simulink model "PandID"  (R2019b)
settings: Solver=VariableStepAuto  StartTime=0.0  StopTime=50  RelTol=1e-3
values from neighbouring files (symbols this model uses):
  L_area = 1    [AFCP_sim.m]
  P_area = 1    [AFCP_sim.m]
  PressureUnit = 1/6894.76    (= 0.000145037680789)    [AFCP_sim.m]
  R_area = 1    [AFCP_sim.m]
  Valve_signal_Unit = 0.00064516    [AFCP_sim.m]
libraries: fl_lib x96, nesl_utility x62, SimscapeFluids_lib x15, simulink x4
(part 1 of 2)
settings Model: OrderedModelArguments=off  Creator=abhig  LastModifiedBy=abhig
settings SFSimCC: SimUserSources=init.c main.c seq.c  SimParseCustomCode=off
settings SFSimCC: SimCustomHeaderCode=|
  | #include "headers.h"
  | #include "init.h"
  | #include "macros.h"
  | #include "seq.h"
settings SFSimCC: SimUserIncludeDirs=|
  | C:\Users\abhig\OneDrive\Desktop\simulation\AFCP_SIMULINK\simulink_test\flightCode\src
  | 
  | C:\Users\abhig\OneDrive\Desktop\simulation\AFCP_SIMULINK\simulink_test\flightCode\include

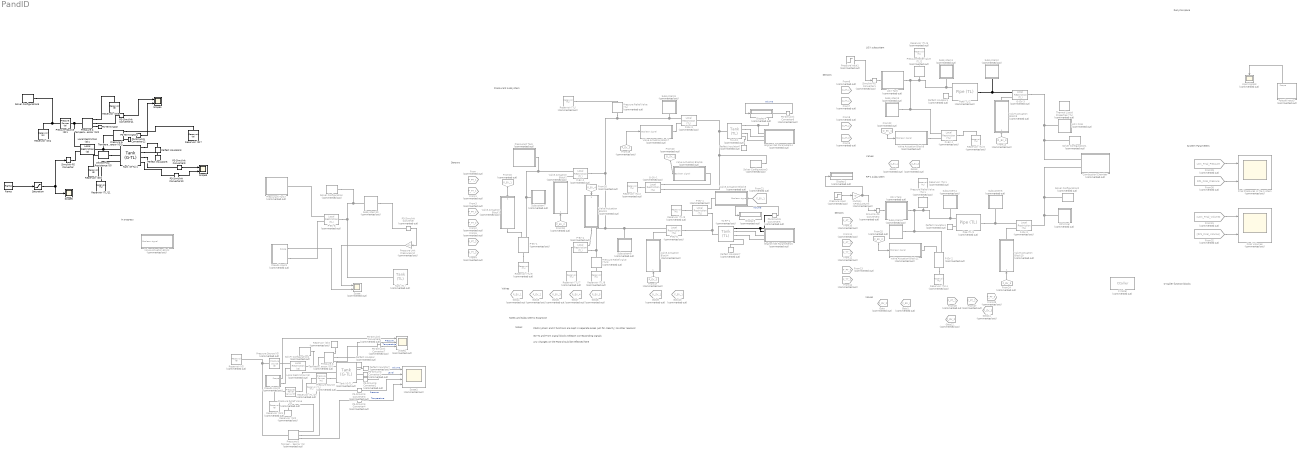
== system PandID ==
  note: System Parameters
  note: In progress
  note: Sensors
  note: Valves
  note: Valves
  note: Sensors
  note: Valves
  note: Sensors
  note: P&ID system and C functions are kept in seperate areas just for clearity; No other reasons!
  note: Notes:
  note: Recycle space
  note: Notes and Subsystems expansion
  note: RP-1 subsystem
  note: Pressurant subsystem
  note: LOX subsystem
  note: C-Caller function blocks
  note: Go-To and From signal blocks teleport corresponding signals
  note: Any changes on the P&ID should be reflected here
  C Caller : CCaller  Commented=on  FunctionName=init  PortSpecificationStruct="%)30     .    , (   8    (     @         %    \"     $    !     0         %  0 \"0    $    _    07)G3F%M90  4&]R=$YA;64 4V-O<&4     26YD97@     5'EP90      4VEZ90      27-';&]B86P   X   !     !@    @    $          4    (     0    D    !         !     )    9FEL95]N86UE          X   !     !@    @    $          4    (     0    D    !         !     )    9FEL95]N86UE          X    X    !@    @    $          4    (     0    8    !         !     &    3W5T<'5T   .    .     8    (    !@         %    \"     $    !     0         )    \"               #@   #     &    \"     0         !0    @    !    !     $         $  $ &EN=#@.    ,     8    (    !          %    \"     $    \"     0         0  ( +3$   X    P    !@    @    ) @        4    (     0    $    !          (  0"
  Combustion Chamber : Subsystem  Commented=on
      mask Display: image('$imagefile'); % Use "Edit Image" on toolstrip to change.
  Display1 : Display  Commented=on
  Display4 : Display  Commented=on
  Display5 : Display  Commented=on
  Engine Inlet Parameters4 : Subsystem  Commented=on
  Engine Inlet Parameters5 : Subsystem  Commented=on
  F-EV-1 : fl_lib/Thermal Liquid/Elements/Local Restriction (TL)  Commented=on  restriction_type=foundation.enum.restriction_type.variable  restriction_area=0.001 m^2  min_area=1e-5 m^2  max_area=0.005 m^2  area=0.01 m^2  Cd=0.64  pressure_recovery=simscape.enum.onoff.on  Re_c=12
      settings: SourceProductName=Simscape  SourceProductBaseCode=SS  InternalSimscapePortConfiguration="{\"Bottom\":[],\"Left\":[{\"id\":\"A\",\"label\":\"A\",\"type\":\"foundation.thermal_liquid.thermal_liquid\"},{\"id\":\"area_in\",\"label\":\"AR\",\"type\":\"input\"}],\"Right\":[{\"id\":\"B\",\"label\":\"B\",\"type\":\"foundation.thermal_liquid.thermal_liquid\"}],\"Top\":[]}"
  F-EV-2 : fl_lib/Thermal Liquid/Elements/Local Restriction (TL)  Commented=on  restriction_type=foundation.enum.restriction_type.variable  restriction_area=0.001 m^2  min_area=R_area*0.01 in^2  max_area=R_area*0.99 in^2  area=R_area in^2  Cd=0.64  pressure_recovery=simscape.enum.onoff.on  Re_c=12
      settings: SourceProductName=Simscape  SourceProductBaseCode=SS  InternalSimscapePortConfiguration="{\"Bottom\":[],\"Left\":[{\"id\":\"A\",\"label\":\"A\",\"type\":\"foundation.thermal_liquid.thermal_liquid\"},{\"id\":\"area_in\",\"label\":\"AR\",\"type\":\"input\"}],\"Right\":[{\"id\":\"B\",\"label\":\"B\",\"type\":\"foundation.thermal_liquid.thermal_liquid\"}],\"Top\":[]}"
  F-EV-3 : fl_lib/Thermal Liquid/Elements/Local Restriction (TL)  Commented=on  restriction_type=foundation.enum.restriction_type.variable  restriction_area=0.001 m^2  min_area=1e-5 in^2  max_area=R_area/2 in^2  area=R_area in^2  Cd=0.64  pressure_recovery=simscape.enum.onoff.on  Re_c=12
      settings: SourceProductName=Simscape  SourceProductBaseCode=SS  InternalSimscapePortConfiguration="{\"Bottom\":[],\"Left\":[{\"id\":\"A\",\"label\":\"A\",\"type\":\"foundation.thermal_liquid.thermal_liquid\"},{\"id\":\"area_in\",\"label\":\"AR\",\"type\":\"input\"}],\"Right\":[{\"id\":\"B\",\"label\":\"B\",\"type\":\"foundation.thermal_liquid.thermal_liquid\"}],\"Top\":[]}"
  Final Pressures in the system : Scope  Commented=on  NumInputPorts=2
  Final Volumes : Scope  Commented=on  NumInputPorts=2
  From : From  Commented=on  GotoTag=P_PT_1  TagVisibility=global
  From1 : From  Commented=on  GotoTag=P_TT_1  TagVisibility=global
  From10 : From  Commented=on  GotoTag=F_PT_1  TagVisibility=global
  From11 : From  Commented=on  GotoTag=F_PT_2  TagVisibility=global
  From12 : From  Commented=on  GotoTag=F_TT_2  TagVisibility=global
  From13 : From  Commented=on  GotoTag=F_PT_3  TagVisibility=global
  From14 : From  Commented=on  GotoTag=F_TT_3  TagVisibility=global
  From15 : From  Commented=on  GotoTag=P_EV_1  TagVisibility=global
  From16 : From  Commented=on  GotoTag=P_EV_4  TagVisibility=global
  From17 : From  Commented=on  GotoTag=P_EV_5  TagVisibility=global
  From18 : From  Commented=on  GotoTag=P_EV_2  TagVisibility=global
  From19 : From  Commented=on  GotoTag=P_EV_3  TagVisibility=global
  From2 : From  Commented=on  GotoTag=P_TT_2  TagVisibility=global
  From20 : From  Commented=on  GotoTag=O_SV_1  TagVisibility=global
  From21 : From  Commented=on  GotoTag=F_EV_1  TagVisibility=global
  From22 : From  Commented=on  GotoTag=O_EV_1  TagVisibility=global
  From23 : From  Commented=on  GotoTag=O_EV_3  TagVisibility=global
  From24 : From  Commented=on  GotoTag=F_EV_3  TagVisibility=global
  From25 : From  Commented=on  GotoTag=F_EV_2  TagVisibility=global
  From26 : From  Commented=on  GotoTag=F_PT_1  TagVisibility=global
  From27 : From  Commented=on  GotoTag=F_PT_2  TagVisibility=global
  From28 : From  Commented=on  GotoTag=F_PT_3  TagVisibility=global
  From29 : From  Commented=on  GotoTag=LOX_Final_Pressure
  From3 : From  Commented=on  GotoTag=P_PT_2  TagVisibility=global
  From30 : From  Commented=on  GotoTag=RP1_Final_Pressure
  From31 : From  Commented=on  GotoTag=LOX_Final_Volume
  From32 : From  Commented=on  GotoTag=RP1_Final_Volume
  From4 : From  Commented=on  GotoTag=P_TT_3  TagVisibility=global
  From5 : From  Commented=on  GotoTag=P_PT_3  TagVisibility=global
  From6 : From  Commented=on  GotoTag=O_PT_1  TagVisibility=global
  From7 : From  Commented=on  GotoTag=O_TT_1  TagVisibility=global
  From8 : From  Commented=on  GotoTag=O_PT_2  TagVisibility=global
  From9 : From  Commented=on  GotoTag=O_PT_3  TagVisibility=global
  Goto : Goto  Commented=on  GotoTag=F_EV_2  TagVisibility=global
  Goto1 : Goto  Commented=on  GotoTag=F_EV_3  TagVisibility=global
  Goto10 : Goto  Commented=on  GotoTag=F_EV_1  TagVisibility=global
  Goto11 : Goto  Commented=on  GotoTag=F_EV_3  TagVisibility=global
  Goto12 : Goto  Commented=on  GotoTag=F_EV_2  TagVisibility=global
  Goto2 : Goto  Commented=on  GotoTag=O_EV_1  TagVisibility=global
  Goto3 : Goto  Commented=on  GotoTag=O_EV_3  TagVisibility=global
  Goto4 : Goto  Commented=on  GotoTag=P_EV_1  TagVisibility=global
  Goto5 : Goto  Commented=on  GotoTag=P_EV_2  TagVisibility=global
  Goto6 : Goto  Commented=on  GotoTag=P_EV_3  TagVisibility=global
  Goto7 : Goto  Commented=on  GotoTag=P_EV_4  TagVisibility=global
  Goto8 : Goto  Commented=on  GotoTag=P_EV_5  TagVisibility=global
  Goto9 : Goto  Commented=on  GotoTag=O_SV_1  TagVisibility=global
  Infinite Flow Resistance (G) : fl_lib/Gas/Elements/Infinite Flow Resistance (G)  p_specify=off  p_priority=None  p=0 MPa  p_nominal_specify=off  p_nominal_unit=MPa  p_nominal_value=1  T_specify=off  T_priority=None  T=0 K  T_nominal_specify=off  T_nominal_unit=K  T_nominal_value=1
      settings: SourceProductName=Simscape  SourceProductBaseCode=SS  InternalSimscapePortConfiguration="{\"Bottom\":[],\"Left\":[{\"id\":\"A\",\"label\":\"A\",\"type\":\"foundation.gas.gas\"}],\"Right\":[{\"id\":\"B\",\"label\":\"B\",\"type\":\"foundation.gas.gas\"}],\"Top\":[]}"
  Input signal3 : Scope  Commented=on
  LOX Final : Subsystem  Commented=on
      mask Display: image('$imagefile'); % Use "Edit Image" on toolstrip to change.
  LOX Tank : Subsystem  Commented=on
      mask Display: image('$imagefile'); % Use "Edit Image" on toolstrip to change.
  Local Restriction (G) : fl_lib/Gas/Elements/Local Restriction (G)  Commented=on  restriction_type=foundation.enum.restriction_type.variable  restriction_area=1e-3 m^2  min_area=1e-10 m^2  max_area=0.005 m^2  area=0.01 m^2  Cd=0.64  B_lam=0.999
      settings: SourceProductName=Simscape  SourceProductBaseCode=SS  InternalSimscapePortConfiguration="{\"Bottom\":[],\"Left\":[{\"id\":\"A\",\"label\":\"A\",\"type\":\"foundation.gas.gas\"},{\"id\":\"area_in\",\"label\":\"AR\",\"type\":\"input\"}],\"Right\":[{\"id\":\"B\",\"label\":\"B\",\"type\":\"foundation.gas.gas\"}],\"Top\":[]}"
  Local Restriction (G)1 : fl_lib/Gas/Elements/Local Restriction (G)  restriction_type=foundation.enum.restriction_type.variable  restriction_area=1e-3 m^2  min_area=1e-10 m^2  max_area=0.005 m^2  area=0.01 m^2  Cd=0.64  B_lam=0.999
      settings: SourceProductName=Simscape  SourceProductBaseCode=SS  InternalSimscapePortConfiguration="{\"Bottom\":[],\"Left\":[{\"id\":\"A\",\"label\":\"A\",\"type\":\"foundation.gas.gas\"},{\"id\":\"area_in\",\"label\":\"AR\",\"type\":\"input\"}],\"Right\":[{\"id\":\"B\",\"label\":\"B\",\"type\":\"foundation.gas.gas\"}],\"Top\":[]}"
  Multiply : Gain  Commented=on  Gain=1/PressureUnit
  O-EV-1 : fl_lib/Thermal Liquid/Elements/Local Restriction (TL)  Commented=on  restriction_type=foundation.enum.restriction_type.variable  restriction_area=0.001 m^2  min_area=1e-5 m^2  max_area=0.005 m^2  area=L_area in^2  Cd=0.64  pressure_recovery=simscape.enum.onoff.on  Re_c=12
      settings: SourceProductName=Simscape  SourceProductBaseCode=SS  InternalSimscapePortConfiguration="{\"Bottom\":[],\"Left\":[{\"id\":\"A\",\"label\":\"A\",\"type\":\"foundation.thermal_liquid.thermal_liquid\"},{\"id\":\"area_in\",\"label\":\"AR\",\"type\":\"input\"}],\"Right\":[{\"id\":\"B\",\"label\":\"B\",\"type\":\"foundation.thermal_liquid.thermal_liquid\"}],\"Top\":[]}"
  O-EV-3 : fl_lib/Thermal Liquid/Elements/Local Restriction (TL)  Commented=on  restriction_type=foundation.enum.restriction_type.variable  restriction_area=0.001 m^2  min_area=1e-5 m^2  max_area=0.005 m^2  area=L_area in^2  Cd=0.64  pressure_recovery=simscape.enum.onoff.on  Re_c=12
      settings: SourceProductName=Simscape  SourceProductBaseCode=SS  InternalSimscapePortConfiguration="{\"Bottom\":[],\"Left\":[{\"id\":\"A\",\"label\":\"A\",\"type\":\"foundation.thermal_liquid.thermal_liquid\"},{\"id\":\"area_in\",\"label\":\"AR\",\"type\":\"input\"}],\"Right\":[{\"id\":\"B\",\"label\":\"B\",\"type\":\"foundation.thermal_liquid.thermal_liquid\"}],\"Top\":[]}"
  O-SV-1 : fl_lib/Thermal Liquid/Elements/Local Restriction (TL)  Commented=on  restriction_type=foundation.enum.restriction_type.variable  restriction_area=0.001 m^2  min_area=1e-5 m^2  max_area=0.005 m^2  area=P_area in^2  Cd=0.64  pressure_recovery=simscape.enum.onoff.on  Re_c=12
      settings: SourceProductName=Simscape  SourceProductBaseCode=SS  InternalSimscapePortConfiguration="{\"Bottom\":[],\"Left\":[{\"id\":\"A\",\"label\":\"A\",\"type\":\"foundation.thermal_liquid.thermal_liquid\"},{\"id\":\"area_in\",\"label\":\"AR\",\"type\":\"input\"}],\"Right\":[{\"id\":\"B\",\"label\":\"B\",\"type\":\"foundation.thermal_liquid.thermal_liquid\"}],\"Top\":[]}"
  P-EV-{1..5} (5 alike) : fl_lib/Thermal Liquid/Elements/Local Restriction (TL)  Commented=on  restriction_type=foundation.enum.restriction_type.variable  restriction_area=0.001 m^2  min_area=1e-5 m^2  max_area=0.005 m^2  area=P_area in^2  Cd=0.64  pressure_recovery=simscape.enum.onoff.on  Re_c=12
      settings: SourceProductName=Simscape  SourceProductBaseCode=SS  InternalSimscapePortConfiguration="{\"Bottom\":[],\"Left\":[{\"id\":\"A\",\"label\":\"A\",\"type\":\"foundation.thermal_liquid.thermal_liquid\"},{\"id\":\"area_in\",\"label\":\"AR\",\"type\":\"input\"}],\"Right\":[{\"id\":\"B\",\"label\":\"B\",\"type\":\"foundation.thermal_liquid.thermal_liquid\"}],\"Top\":[]}"
  P-EV-6 : fl_lib/Thermal Liquid/Elements/Local Restriction (TL)  Commented=on  restriction_type=foundation.enum.restriction_type.variable  restriction_area=0.001 m^2  min_area=P_area*0.01 in^2  max_area=P_area*0.99 in^2  area=P_area in^2  Cd=0.64  pressure_recovery=simscape.enum.onoff.on  Re_c=12
      settings: SourceProductName=Simscape  SourceProductBaseCode=SS  InternalSimscapePortConfiguration="{\"Bottom\":[],\"Left\":[{\"id\":\"A\",\"label\":\"A\",\"type\":\"foundation.thermal_liquid.thermal_liquid\"},{\"id\":\"area_in\",\"label\":\"AR\",\"type\":\"input\"}],\"Right\":[{\"id\":\"B\",\"label\":\"B\",\"type\":\"foundation.thermal_liquid.thermal_liquid\"}],\"Top\":[]}"
  PS Terminator : fl_lib/Physical Signals/Sinks/PS Terminator
      settings: SourceProductName=Simscape
  PS Terminator1 : fl_lib/Physical Signals/Sinks/PS Terminator
      settings: SourceProductName=Simscape
  PS-Simulink Converter{,1..8} (9 alike) : nesl_utility/PS-Simulink Converter  Commented=on  PhysicalDomain=network_engine_domain  SubClassName=ps_output  LeftPortType=input  RightPortType=output  PseudoPeriodic=off  Frequencies=[]  Unit=inherit  AffineConversion=off
  PS-Simulink Converter{9..12} (4 alike) : nesl_utility/PS-Simulink Converter  PhysicalDomain=network_engine_domain  SubClassName=ps_output  LeftPortType=input  RightPortType=output  PseudoPeriodic=off  Frequencies=[]  Unit=inherit  AffineConversion=off
  Perfect Insulator{,1..2,4,6..7} (6 alike) : fl_lib/Thermal/Thermal Elements/Perfect Insulator  Commented=on  T_specify=off  T_priority=None  T=0 K  T_nominal_specify=off  T_nominal_unit=K  T_nominal_value=1
      settings: SourceProductName=Simscape
  Perfect Insulator3 : fl_lib/Thermal/Thermal Elements/Perfect Insulator  T_specify=off  T_priority=None  T=0 K  T_nominal_specify=off  T_nominal_unit=K  T_nominal_value=1
      settings: SourceProductName=Simscape
  Perfect Insulator5 : fl_lib/Thermal/Thermal Elements/Perfect Insulator  T_specify=off  T_priority=None  T=0 K  T_nominal_specify=off  T_nominal_unit=K  T_nominal_value=1
      settings: SourceProductName=Simscape
  Pipe (TL)1 : SimscapeFluids_lib/Thermal Liquid/Pipes & Fittings/Pipe (TL)  Commented=on  dynamic_compressibility=1  inertia=0  num_segments=1  pipe_length=5 m  area=R_area in^2  Dh=0.1128 m  wall_spec=1  Dh_rigid=0.1128 m  wall_compliance=1.2e-6 m/MPa  wall_time_constant=0.01 s  elevation_gain=0 m  g=9.81 m/s^2  pressure_loss_spec=1  length_add=1 m  roughness=1.5e-5 m  Re_friction_TLU=[ 400 1000 1.5e+3 3e+3 4e+3 6e+3 1e+4 2e+4 4e+4 6e+4 1e+5 1e+8 ]  friction_factor_TLU=[ 0.264 0.112 0.07099999999999999 0.0417 0.0387 0.0268 0.025 0.0232 0.0226 0.022 0.0214 0.0214 ]  shape_factor=64  mdot_nominal=[ 0.1 1 ] kg/s  p_diff_nominal=[ 0.001 0.01 ] MPa  mdot_threshold=1e-6 kg/s  Re_lam=2e+3  Re_tur=4e+3  heat_transfer_spec=1  mdot_nominal_heat=[ 0.1 1 ] kg/s  T_in_nominal=[ 293.15 293.15 ] K  T_out_nominal=[ 300 300 ] K  p_in_nominal_heat=[ 0.101325 0.101325 ] MPa  T_wall_nominal=[ 303.15 303.15 ] K  a_coeff=0.023  b_Re_power=0.8  c_Pr_power=0.4  Nu_lam=3.66  Re_Colburn_TLU=[ 100 150 1000 ]  Colburn_factor_TLU=[ 0.019 0.013 0.002 ]  Re_Nu_TLU=[ 100 150 1000 ]  Pr_Nu_TLU=[ 1 10 ]  Nu_TLU=[ 3.72 4.21; 3.75 4.44; 4.21 7.15 ]  T0_vec=293.15 K  p0_vec=0.101325 MPa  mdot0=0.1 kg/s
      settings: SourceProductName=Simscape Fluids  SourceProductBaseCode=SH
  Pipe (TL)2 : SimscapeFluids_lib/Thermal Liquid/Pipes & Fittings/Pipe (TL)  Commented=on  dynamic_compressibility=1  inertia=0  num_segments=1  pipe_length=5 m  area=L_area in^2  Dh=0.1128 m  wall_spec=1  Dh_rigid=0.1128 m  wall_compliance=1.2e-6 m/MPa  wall_time_constant=0.01 s  elevation_gain=0 m  g=9.81 m/s^2  pressure_loss_spec=1  length_add=1 m  roughness=1.5e-5 m  Re_friction_TLU=[ 400 1000 1.5e+3 3e+3 4e+3 6e+3 1e+4 2e+4 4e+4 6e+4 1e+5 1e+8 ]  friction_factor_TLU=[ 0.264 0.112 0.07099999999999999 0.0417 0.0387 0.0268 0.025 0.0232 0.0226 0.022 0.0214 0.0214 ]  shape_factor=64  mdot_nominal=[ 0.1 1 ] kg/s  p_diff_nominal=[ 0.001 0.01 ] MPa  mdot_threshold=1e-6 kg/s  Re_lam=2e+3  Re_tur=4e+3  heat_transfer_spec=1  mdot_nominal_heat=[ 0.1 1 ] kg/s  T_in_nominal=[ 293.15 293.15 ] K  T_out_nominal=[ 300 300 ] K  p_in_nominal_heat=[ 0.101325 0.101325 ] MPa  T_wall_nominal=[ 303.15 303.15 ] K  a_coeff=0.023  b_Re_power=0.8  c_Pr_power=0.4  Nu_lam=3.66  Re_Colburn_TLU=[ 100 150 1000 ]  Colburn_factor_TLU=[ 0.019 0.013 0.002 ]  Re_Nu_TLU=[ 100 150 1000 ]  Pr_Nu_TLU=[ 1 10 ]  Nu_TLU=[ 3.72 4.21; 3.75 4.44; 4.21 7.15 ]  T0_vec=293.15 K  p0_vec=0.101325 MPa  mdot0=0.1 kg/s
      settings: SourceProductName=Simscape Fluids  SourceProductBaseCode=SH
  Pressurant Tank : Subsystem  Commented=on
      mask Display: image('$imagefile'); % Use "Edit Image" on toolstrip to change.
  Pressurant Tank1 : Subsystem  Commented=on
      mask Display: image('$imagefile'); % Use "Edit Image" on toolstrip to change.
  Pressure & Temperature Sensor (G) : fl_lib/Gas/Sensors/Pressure & Temperature Sensor (G)  Commented=on
      settings: SourceProductName=Simscape  SourceProductBaseCode=SS  InternalSimscapePortConfiguration="{\"Bottom\":[],\"Left\":[{\"id\":\"A\",\"label\":\"A\",\"type\":\"foundation.gas.gas\"}],\"Right\":[{\"id\":\"B\",\"label\":\"B\",\"type\":\"foundation.gas.gas\"},{\"id\":\"P\",\"label\":\"P\",\"type\":\"output\"},{\"id\":\"T\",\"label\":\"T\",\"type\":\"output\"}],\"Top\":[]}"
  Pressure & Temperature Sensor (G)1 : fl_lib/Gas/Sensors/Pressure & Temperature Sensor (G)  Commented=on
      settings: SourceProductName=Simscape  SourceProductBaseCode=SS  InternalSimscapePortConfiguration="{\"Bottom\":[],\"Left\":[{\"id\":\"A\",\"label\":\"A\",\"type\":\"foundation.gas.gas\"}],\"Right\":[{\"id\":\"B\",\"label\":\"B\",\"type\":\"foundation.gas.gas\"},{\"id\":\"P\",\"label\":\"P\",\"type\":\"output\"},{\"id\":\"T\",\"label\":\"T\",\"type\":\"output\"}],\"Top\":[]}"
  Pressure & Temperature Sensor (G)2 : fl_lib/Gas/Sensors/Pressure & Temperature Sensor (G)
      settings: SourceProductName=Simscape  SourceProductBaseCode=SS  InternalSimscapePortConfiguration="{\"Bottom\":[],\"Left\":[{\"id\":\"A\",\"label\":\"A\",\"type\":\"foundation.gas.gas\"}],\"Right\":[{\"id\":\"B\",\"label\":\"B\",\"type\":\"foundation.gas.gas\"},{\"id\":\"P\",\"label\":\"P\",\"type\":\"output\"},{\"id\":\"T\",\"label\":\"T\",\"type\":\"output\"}],\"Top\":[]}"
  Pressure & Temperature Sensor (G)3 : fl_lib/Gas/Sensors/Pressure & Temperature Sensor (G)
      settings: SourceProductName=Simscape  SourceProductBaseCode=SS  InternalSimscapePortConfiguration="{\"Bottom\":[],\"Left\":[{\"id\":\"A\",\"label\":\"A\",\"type\":\"foundation.gas.gas\"}],\"Right\":[{\"id\":\"B\",\"label\":\"B\",\"type\":\"foundation.gas.gas\"},{\"id\":\"P\",\"label\":\"P\",\"type\":\"output\"},{\"id\":\"T\",\"label\":\"T\",\"type\":\"output\"}],\"Top\":[]}"
  Pressure Relief Valve (G) : SimscapeFluids_lib/Gas/Valves & Orifices/Pressure Control Valves/Pressure Relief Valve (G)  Commented=on  pressure_spec=fluids.gas.enum.pressure_control_spec.dp  p_set_gauge=0.1 MPa  p_set_differential=0 MPa  p_range=0.1 MPa  iso_cond_spec=fluids.gas.enum.iso_cond_spec.conductance  iso_opening_spec=fluids.gas.enum.iso_opening_spec.linear  C_max=1.6 l/s/bar  C_min=1e-5 l/s/bar  B_crit=0.3  p_control_C_TLU=[0.2 : 0.2 : 1.2] MPa  C_TLU=[1e-05, .32, .64, .96, 1.28, 1.6] l/s/bar  B_crit_TLU=0.3 * ones(1, 6)  m=0.5  Cv_max=0.4  Cv_min=1e-6  p_control_Cv_TLU=[0.2 : 0.2 : 1.2] MPa  Cv_TLU=[1e-06, .08, .16, .24, .32, .4]  Kv_max=0.3  Kv_min=1e-6  p_control_Kv_TLU=[0.2 : 0.2 : 1.2] MPa  Kv_TLU=[1e-06, .06, .12, .18, .24, .3]  area_max=1e-4 m^2  area_leak=1e-12 m^2  p_control_area_TLU=[0.2 : 0.2 : 1.2] MPa  restriction_area_TLU=[1e-10, 2e-06, 4e-06, 6e-06, 8e-06, 1e-05] m^2  area=0.01 m^2  smoothing_factor=0  B_lam=0.999  T0=293.15 K  rho0=1.185 kg/m^3
      settings: SourceProductName=Simscape Fluids  SourceProductBaseCode=SH  InternalSimscapePortConfiguration="{\"Bottom\":[],\"Left\":[{\"id\":\"A\",\"label\":\"A\",\"type\":\"foundation.gas.gas\"}],\"Right\":[{\"id\":\"B\",\"label\":\"B\",\"type\":\"foundation.gas.gas\"}],\"Top\":[]}"
  Pressure Relief Valve (TL) : SimscapeFluids_lib/Thermal Liquid/Valves & Orifices/Pressure Control Valves/Pressure Relief Valve (TL)  Commented=on  pressure_spec=1  p_set_gauge=0.1 MPa  p_set_differential=0 MPa  p_range=0.15 MPa  area_max=1e-4 m^2  area_leak=1e-12 m^2  smoothing_factor=0.01  area=0.01 m^2  length=0.1 m  Cd=0.7  Re_c=12  mdot_A_specify=off  mdot_A_priority=None  mdot_A=1 kg/s  mdot_A_nominal_specify=off  mdot_A_nominal_unit=kg/s  mdot_A_nominal_value=1
      settings: SourceProductName=Simscape Fluids  SourceProductBaseCode=SH  InternalSimscapePortConfiguration="{\"Bottom\":[],\"Left\":[{\"id\":\"A\",\"label\":\"A\",\"type\":\"foundation.thermal_liquid.thermal_liquid\"}],\"Right\":[{\"id\":\"B\",\"label\":\"B\",\"type\":\"foundation.thermal_liquid.thermal_liquid\"}],\"Top\":[]}"
  Pressure Relief Valve (TL)1 : SimscapeFluids_lib/Thermal Liquid/Valves & Orifices/Pressure Control Valves/Pressure Relief Valve (TL)  Commented=on  pressure_spec=1  p_set_gauge=0.1 psi  p_set_differential=0 MPa  p_range=0.15 psi  area_max=R_area/10 in^2  area_leak=1e-6 in^2  smoothing_factor=0.01  area=R_area in^2  length=0.1 m  Cd=0.7  Re_c=12  mdot_A_specify=off  mdot_A_priority=None  mdot_A=1 kg/s  mdot_A_nominal_specify=off  mdot_A_nominal_unit=kg/s  mdot_A_nominal_value=1
      settings: SourceProductName=Simscape Fluids  SourceProductBaseCode=SH  InternalSimscapePortConfiguration="{\"Bottom\":[],\"Left\":[{\"id\":\"A\",\"label\":\"A\",\"type\":\"foundation.thermal_liquid.thermal_liquid\"}],\"Right\":[{\"id\":\"B\",\"label\":\"B\",\"type\":\"foundation.thermal_liquid.thermal_liquid\"}],\"Top\":[]}"
  Pressure Relief Valve (TL)2 : SimscapeFluids_lib/Thermal Liquid/Valves & Orifices/Pressure Control Valves/Pressure Relief Valve (TL)  Commented=on  pressure_spec=1  p_set_gauge=0.1 MPa  p_set_differential=0 MPa  p_range=0.15 MPa  area_max=1e-4 m^2  area_leak=1e-12 m^2  smoothing_factor=0.01  area=0.01 m^2  length=0.1 m  Cd=0.7  Re_c=12  mdot_A_specify=off  mdot_A_priority=None  mdot_A=1 kg/s  mdot_A_nominal_specify=off  mdot_A_nominal_unit=kg/s  mdot_A_nominal_value=1
      settings: SourceProductName=Simscape Fluids  SourceProductBaseCode=SH  InternalSimscapePortConfiguration="{\"Bottom\":[],\"Left\":[{\"id\":\"A\",\"label\":\"A\",\"type\":\"foundation.thermal_liquid.thermal_liquid\"}],\"Right\":[{\"id\":\"B\",\"label\":\"B\",\"type\":\"foundation.thermal_liquid.thermal_liquid\"}],\"Top\":[]}"
  Pressure Relief Valve (TL)3 : SimscapeFluids_lib/Thermal Liquid/Valves & Orifices/Pressure Control Valves/Pressure Relief Valve (TL)  Commented=on  pressure_spec=1  p_set_gauge=0.1 MPa  p_set_differential=0 MPa  p_range=0.15 MPa  area_max=1e-4 m^2  area_leak=1e-12 m^2  smoothing_factor=0.01  area=0.01 m^2  length=0.1 m  Cd=0.7  Re_c=12  mdot_A_specify=off  mdot_A_priority=None  mdot_A=1 kg/s  mdot_A_nominal_specify=off  mdot_A_nominal_unit=kg/s  mdot_A_nominal_value=1
      settings: SourceProductName=Simscape Fluids  SourceProductBaseCode=SH  InternalSimscapePortConfiguration="{\"Bottom\":[],\"Left\":[{\"id\":\"A\",\"label\":\"A\",\"type\":\"foundation.thermal_liquid.thermal_liquid\"}],\"Right\":[{\"id\":\"B\",\"label\":\"B\",\"type\":\"foundation.thermal_liquid.thermal_liquid\"}],\"Top\":[]}"
  Pressure Source (G) : fl_lib/Gas/Sources/Pressure Source (G)  Commented=on  power_spec=foundation.enum.power_spec.isentropic  pressure_differential=15 MPa  area_A=0.01 m^2  area_B=0.01 m^2
      settings: SourceProductName=Simscape  SourceProductBaseCode=SS  InternalSimscapePortConfiguration="{\"Bottom\":[],\"Left\":[{\"id\":\"A\",\"label\":\"A\",\"type\":\"foundation.gas.gas\"}],\"Right\":[{\"id\":\"B\",\"label\":\"B\",\"type\":\"foundation.gas.gas\"}],\"Top\":[]}"
  Pressure Source (G)1 : fl_lib/Gas/Sources/Pressure Source (G)  power_spec=foundation.enum.power_spec.isentropic  pressure_differential=10 MPa  area_A=0.01 m^2  area_B=0.01 m^2
      settings: SourceProductName=Simscape  SourceProductBaseCode=SS  InternalSimscapePortConfiguration="{\"Bottom\":[],\"Left\":[{\"id\":\"A\",\"label\":\"A\",\"type\":\"foundation.gas.gas\"}],\"Right\":[{\"id\":\"B\",\"label\":\"B\",\"type\":\"foundation.gas.gas\"}],\"Top\":[]}"
  Pressure Source (TL) : fl_lib/Thermal Liquid/Sources/Pressure Source (TL)  Commented=on  commanded_pressure=10 MPa  area=0.01 m^2
      settings: SourceProductName=Simscape  SourceProductBaseCode=SS  InternalSimscapePortConfiguration="{\"Bottom\":[],\"Left\":[{\"id\":\"A\",\"label\":\"A\",\"type\":\"foundation.thermal_liquid.thermal_liquid\"}],\"Right\":[{\"id\":\"B\",\"label\":\"B\",\"type\":\"foundation.thermal_liquid.thermal_liquid\"}],\"Top\":[]}"
  Pressure Unit : Gain  Commented=on  Gain=PressureUnit
  Pressure input : Step  Commented=on  Time=50  After=1000  SampleTime=0
  Pressure input1 : Step  Commented=on  Time=5  After=1000000  SampleTime=0
  Pseudo input1 : Subsystem  Commented=on
  Pseudo input2 : Subsystem  Commented=on
  Pseudo input3 : Subsystem  Commented=on
  RP-1 Tank : Subsystem  Commented=on
      mask Display: image('$imagefile'); % Use "Edit Image" on toolstrip to change.
  RP1 Final : Subsystem  Commented=on
      mask Display: image('$imagefile'); % Use "Edit Image" on toolstrip to change.
  Ramp : simulink/Sources/Ramp  slope=0.0005  start=30  InitialOutput=0
  Reservoir (G){,1..3} (4 alike) : fl_lib/Gas/Elements/Reservoir (G)  Commented=on  pressure_spec=foundation.enum.pressure_spec.atmospheric  reservoir_pressure=0.101325 MPa  reservoir_temperature=293.15 K  area_A=0.01 m^2
      settings: SourceProductName=Simscape  SourceProductBaseCode=SS
  Reservoir (G)4 : fl_lib/Gas/Elements/Reservoir (G)  pressure_spec=foundation.enum.pressure_spec.specified  reservoir_pressure=20 MPa  reservoir_temperature=293.15 K  area_A=0.01 m^2
      settings: SourceProductName=Simscape  SourceProductBaseCode=SS
  Reservoir (G)5 : fl_lib/Gas/Elements/Reservoir (G)  pressure_spec=foundation.enum.pressure_spec.atmospheric  reservoir_pressure=0.101325 MPa  reservoir_temperature=293.15 K  area_A=0.01 m^2
      settings: SourceProductName=Simscape  SourceProductBaseCode=SS
  Reservoir (G)6 : fl_lib/Gas/Elements/Reservoir (G)  pressure_spec=foundation.enum.pressure_spec.atmospheric  reservoir_pressure=0.101325 MPa  reservoir_temperature=293.15 K  area_A=0.01 m^2
      settings: SourceProductName=Simscape  SourceProductBaseCode=SS
  Reservoir (G)7 : fl_lib/Gas/Elements/Reservoir (G)  pressure_spec=foundation.enum.pressure_spec.atmospheric  reservoir_pressure=0.101325 MPa  reservoir_temperature=293.15 K  area_A=0.01 m^2
      settings: SourceProductName=Simscape  SourceProductBaseCode=SS
  Reservoir (TL){,2..3,7..9} (6 alike) : fl_lib/Thermal Liquid/Elements/Reservoir (TL)  Commented=on  pressure_spec=foundation.enum.pressure_spec.atmospheric  reservoir_pressure=0.101325 MPa  reservoir_temperature=293.15 K  area=P_area in^2
      settings: SourceProductName=Simscape  SourceProductBaseCode=SS
  Reservoir (TL)1 : fl_lib/Thermal Liquid/Elements/Reservoir (TL)  Commented=on  pressure_spec=foundation.enum.pressure_spec.atmospheric  reservoir_pressure=0.101325 MPa  reservoir_temperature=293.15 K  area=R_area in^2
      settings: SourceProductName=Simscape  SourceProductBaseCode=SS
  Reservoir (TL)10 : fl_lib/Thermal Liquid/Elements/Reservoir (TL)  Commented=on  pressure_spec=foundation.enum.pressure_spec.atmospheric  reservoir_pressure=0.101325 MPa  reservoir_temperature=293.15 K  area=0.01 m^2
      settings: SourceProductName=Simscape  SourceProductBaseCode=SS
  Reservoir (TL)11 : fl_lib/Thermal Liquid/Elements/Reservoir (TL)  pressure_spec=foundation.enum.pressure_spec.atmospheric  reservoir_pressure=5 MPa  reservoir_temperature=293.15 K  area=0.01 m^2
      settings: SourceProductName=Simscape  SourceProductBaseCode=SS
  Reservoir (TL)4 : fl_lib/Thermal Liquid/Elements/Reservoir (TL)  Commented=on  pressure_spec=foundation.enum.pressure_spec.atmospheric  reservoir_pressure=0.101325 MPa  reservoir_temperature=293.15 K  area=R_area in^2
      settings: SourceProductName=Simscape  SourceProductBaseCode=SS
  Reservoir (TL)5 : fl_lib/Thermal Liquid/Elements/Reservoir (TL)  Commented=on  pressure_spec=foundation.enum.pressure_spec.atmospheric  reservoir_pressure=0.101325 MPa  reservoir_temperature=293.15 K  area=L_area in^2
      settings: SourceProductName=Simscape  SourceProductBaseCode=SS
  Reservoir (TL)6 : fl_lib/Thermal Liquid/Elements/Reservoir (TL)  Commented=on  pressure_spec=foundation.enum.pressure_spec.atmospheric  reservoir_pressure=0.101325 MPa  reservoir_temperature=293.15 K  area=L_area in^2
      settings: SourceProductName=Simscape  SourceProductBaseCode=SS
  Saturation : Saturate  UpperLimit=0.003
  Scope : Scope  Commented=on  NumInputPorts=2
  Scope1 : Scope  Commented=on  NumInputPorts=4
  Scope2 : Scope  Commented=on  NumInputPorts=3
  Scope3 : Scope  NumInputPorts=2
  Scope4 : Scope  NumInputPorts=2
  Scope5 : Scope
  Simulink-PS Converter : nesl_utility/Simulink-PS Converter  PhysicalDomain=network_engine_domain  SubClassName=ps_input  LeftPortType=input  RightPortType=output  PseudoPeriodic=off  Frequencies=[]  NoiseDistribution=none  NoiseParameters=[]  Unit=m^2  AffineConversion=off  FilteringAndDerivatives=provide  SimscapeFilterOrder=1  InputFilterTimeConstant=0.001  UdotUserProvided=0
  Simulink-PS Converter1 : nesl_utility/Simulink-PS Converter  Commented=on  PhysicalDomain=network_engine_domain  SubClassName=ps_input  LeftPortType=input  RightPortType=output  PseudoPeriodic=off  Frequencies=[]  NoiseDistribution=none  NoiseParameters=[]  Unit=Pa  AffineConversion=off  FilteringAndDerivatives=provide  SimscapeFilterOrder=1  InputFilterTimeConstant=0.001  UdotUserProvided=0
  Simulink-PS Converter2 : nesl_utility/Simulink-PS Converter  Commented=on  PhysicalDomain=network_engine_domain  SubClassName=ps_input  LeftPortType=input  RightPortType=output  PseudoPeriodic=off  Frequencies=[]  NoiseDistribution=none  NoiseParameters=[]  Unit=Pa  AffineConversion=off  FilteringAndDerivatives=provide  SimscapeFilterOrder=1  InputFilterTimeConstant=0.001  UdotUserProvided=0
  Solver Configuration{,1..4} (5 alike) : nesl_utility/Solver Configuration  Commented=on  PhysicalDomain=network_engine_domain  SubClassName=solver  LeftPortType=input  RightPortType=generic  Tones=[]  Harmonics=[]  SimulateNoise=off  Profile=off  UseLocalSampling=off  EnableSwitchedLinearOptims=on  FrequencyDomain=off  UseCCode=off  RelTol=0.001  AbsTol=1e-06  MinStep=1e-09  ToWorkspace=off  RevertToSquareIcSolve=off  NumHomotopyIterations=100  PhasorMode=off  PhasorModeNumHarmonics=1  DoDC=off  ResidualTolerance=1e-09  UseLocalSolver=off  LocalSolverChoice=NE_BACKWARD_EULER_ADVANCER  LocalSolverSampleTime=0.001  DoFixedCost=off  MaxNonlinIter=3  MaxModeIter=2  LinearAlgebra=auto  EquationFormulation=NE_TIME_EF  DelaysMemoryBudget=1024  AutomaticFiltering=on  FilteringTimeConstant=0.001  PartitionStorageMethod=AS_NEEDED  PartitionMemoryBudget=1024  PartitionMethod=ROBUST
  Solver Configuration5 : nesl_utility/Solver Configuration  PhysicalDomain=network_engine_domain  SubClassName=solver  LeftPortType=input  RightPortType=generic  Tones=[]  Harmonics=[]  SimulateNoise=off  Profile=off  UseLocalSampling=off  EnableSwitchedLinearOptims=on  FrequencyDomain=off  UseCCode=off  RelTol=0.001  AbsTol=1e-06  MinStep=1e-09  ToWorkspace=off  RevertToSquareIcSolve=off  NumHomotopyIterations=100  PhasorMode=off  PhasorModeNumHarmonics=1  DoDC=off  ResidualTolerance=1e-09  UseLocalSolver=off  LocalSolverChoice=NE_BACKWARD_EULER_ADVANCER  LocalSolverSampleTime=0.001  DoFixedCost=off  MaxNonlinIter=3  MaxModeIter=2  LinearAlgebra=auto  EquationFormulation=NE_TIME_EF  DelaysMemoryBudget=1024  AutomaticFiltering=on  FilteringTimeConstant=0.001  PartitionStorageMethod=AS_NEEDED  PartitionMemoryBudget=1024  PartitionMethod=ROBUST
  Subsystem1 : Subsystem  Commented=on
      mask Display: image('$imagefile'); % Use "Edit Image" on toolstrip to change.
  Subsystem10 : Subsystem  Commented=on
      mask Display: image('$imagefile'); % Use "Edit Image" on toolstrip to change.
  Subsystem2 : Subsystem  Commented=on
      mask Display: image('$imagefile'); % Use "Edit Image" on toolstrip to change.
  Subsystem3 : Subsystem  Commented=on
      mask Display: image('$imagefile'); % Use "Edit Image" on toolstrip to change.
  Subsystem4 : Subsystem  Commented=on
      mask Display: image('$imagefile'); % Use "Edit Image" on toolstrip to change.
  Subsystem5 : Subsystem  Commented=on
      mask Display: image('$imagefile'); % Use "Edit Image" on toolstrip to change.
  Subsystem6 : Subsystem  Commented=on
      mask Display: image('$imagefile'); % Use "Edit Image" on toolstrip to change.
  Subsystem7 : Subsystem  Commented=on
      mask Display: image('$imagefile'); % Use "Edit Image" on toolstrip to change.
  Subsystem8 : Subsystem  Commented=on
      mask Display: image('$imagefile'); % Use "Edit Image" on toolstrip to change.
  Subsystem9 : Subsystem  Commented=on
      mask Display: image('$imagefile'); % Use "Edit Image" on toolstrip to change.
  Tank (G-TL) : SimscapeFluids_lib/Fluid Network Interfaces/Tanks & Accumulators/Tank (G-TL)  Commented=on  volume_total=10 m^3  volume_spec=1  tank_area=1 m^2  level_TLU=[0, 3, 5] m  volume_TLU=[0, 4, 6] m^3  inlet_height=0.001 m  inlet_areas_A1B1=[.01, .01] m^2  area_A2=0.01 m^2  g=9.81 m/s^2  p_gas_tank_specify=off  p_gas_tank_priority=High  p_gas_tank=0.101325 MPa  p_gas_tank_nominal_specify=off  p_gas_tank_nominal_unit=MPa  p_gas_tank_nominal_value=1  T_gas_tank_specify=off  T_gas_tank_priority=High  T_gas_tank=293.15 K  T_gas_tank_nominal_specify=off  T_gas_tank_nominal_unit=K  T_gas_tank_nominal_value=1  rho_gas_tank_specify=off  rho_gas_tank_priority=None  rho_gas_tank=1.2 kg/m^3  rho_gas_tank_nominal_specify=off  rho_gas_tank_nominal_unit=kg/m^3  rho_gas_tank_nominal_value=1  T_liquid_tank_specify=off  T_liquid_tank_priority=High  T_liquid_tank=293.15 K  T_liquid_tank_nominal_specify=off  T_liquid_tank_nominal_unit=K  T_liquid_tank_nominal_value=1  level_specify=off  level_priority=High  level=5 m  level_nominal_specify=off  level_nominal_unit=m  level_nominal_value=1  volume_liquid_specify=off  volume_liquid_priority=None  volume_liquid=5 m^3  volume_liquid_nominal_specify=off  volume_liquid_nominal_unit=m^3  volume_liquid_nominal_value=1  mass_liquid_specify=off  mass_liquid_priority=None  mass_liquid=5e+3 kg  mass_liquid_nominal_specify=off  mass_liquid_nominal_unit=kg  mass_liquid_nominal_value=1  inlet_heights_A2B2=[.1, 0] m  inlet_areas_A2B2=[.01, .01] m^2  inlet_heights_A2B2C2=[.1, .05, 0] m  inlet_areas_A2B2C2=[.01, .01, .01] m^2
      settings: SourceProductName=Simscape Fluids  SourceProductBaseCode=SH  InternalSimscapePortConfiguration="{\"Bottom\":[],\"Left\":[{\"id\":\"A1\",\"label\":\"A1\",\"type\":\"foundation.gas.gas\"},{\"id\":\"B1\",\"label\":\"B1\",\"type\":\"foundation.gas.gas\"},{\"id\":\"A2\",\"label\":\"A2\",\"type\":\"foundation.thermal_liquid.thermal_liquid\"}],\"Right\":[{\"id\":\"H1\",\"label\":\"H1\",\"type\":\"foundation.thermal.thermal\"},{\"id\":\"H2\",\"label\":\"H2\",\"type\":\"foundation.thermal.thermal\"},{\"id\":\"V_out\",\"label\":\"V\",\"type\":\"output\"},{\"id\":\"L_out\",\"label\":\"L\",\"type\":\"output\"}],\"Top\":[]}"
  Tank (G-TL)1 : SimscapeFluids_lib/Fluid Network Interfaces/Tanks & Accumulators/Tank (G-TL)  volume_total=1000 m^3  volume_spec=1  tank_area=10 m^2  level_TLU=[0, 3, 5] m  volume_TLU=[0, 4, 6] m^3  inlet_height=0 m  inlet_areas_A1B1=[.01, .01] m^2  area_A2=0.01 m^2  g=9.81 m/s^2  p_gas_tank_specify=off  p_gas_tank_priority=High  p_gas_tank=0.101325 MPa  p_gas_tank_nominal_specify=off  p_gas_tank_nominal_unit=MPa  p_gas_tank_nominal_value=1  T_gas_tank_specify=on  T_gas_tank_priority=High  T_gas_tank=293.15 K  T_gas_tank_nominal_specify=off  T_gas_tank_nominal_unit=K  T_gas_tank_nominal_value=1  rho_gas_tank_specify=off  rho_gas_tank_priority=None  rho_gas_tank=1.2 kg/m^3  rho_gas_tank_nominal_specify=off  rho_gas_tank_nominal_unit=kg/m^3  rho_gas_tank_nominal_value=1  T_liquid_tank_specify=on  T_liquid_tank_priority=High  T_liquid_tank=293.15 K  T_liquid_tank_nominal_specify=off  T_liquid_tank_nominal_unit=K  T_liquid_tank_nominal_value=1  level_specify=on  level_priority=High  level=50 m  level_nominal_specify=off  level_nominal_unit=m  level_nominal_value=1  volume_liquid_specify=on  volume_liquid_priority=None  volume_liquid=50 m^3  volume_liquid_nominal_specify=off  volume_liquid_nominal_unit=m^3  volume_liquid_nominal_value=1  mass_liquid_specify=off  mass_liquid_priority=None  mass_liquid=5e+3 kg  mass_liquid_nominal_specify=off  mass_liquid_nominal_unit=kg  mass_liquid_nominal_value=1  inlet_heights_A2B2=[.1, 0] m  inlet_areas_A2B2=[.01, .01] m^2  inlet_heights_A2B2C2=[.1, .05, 0] m  inlet_areas_A2B2C2=[.01, .01, .01] m^2
      settings: SourceProductName=Simscape Fluids  SourceProductBaseCode=SH  InternalSimscapePortConfiguration="{\"Bottom\":[],\"Left\":[{\"id\":\"A1\",\"label\":\"A1\",\"type\":\"foundation.gas.gas\"},{\"id\":\"B1\",\"label\":\"B1\",\"type\":\"foundation.gas.gas\"},{\"id\":\"A2\",\"label\":\"A2\",\"type\":\"foundation.thermal_liquid.thermal_liquid\"}],\"Right\":[{\"id\":\"H1\",\"label\":\"H1\",\"type\":\"foundation.thermal.thermal\"},{\"id\":\"H2\",\"label\":\"H2\",\"type\":\"foundation.thermal.thermal\"},{\"id\":\"V_out\",\"label\":\"V\",\"type\":\"output\"},{\"id\":\"L_out\",\"label\":\"L\",\"type\":\"output\"}],\"Top\":[]}"
  Tank (TL) : SimscapeFluids_lib/Thermal Liquid/Tanks & Accumulators/Tank (TL)  Commented=on  pressure_spec=1  tank_pressure=0.101325 MPa  max_capacity=10 m^3  volume_spec=1  tank_area=1 m^2  level_TLU=[0, 3, 5] m  volume_TLU=[0, 4, 6] m^3  inlet_height=0.1 in  inlet_area=P_area in^2  g=9.81 m/s^2  level_specify=off  level_priority=High  level=5 m  level_nominal_specify=off  level_nominal_unit=m  level_nominal_value=1  volume_specify=off  volume_priority=None  volume=5 m^3  volume_nominal_specify=off  volume_nominal_unit=m^3  volume_nominal_value=1  mass_specify=off  mass_priority=None  mass=5e+3 kg  mass_nominal_specify=off  mass_nominal_unit=kg  mass_nominal_value=1  T_tank_specify=off  T_tank_priority=High  T_tank=293.15 K  T_tank_nominal_specify=off  T_tank_nominal_unit=K  T_tank_nominal_value=1  inlet_heights_AB=[.1, 0] m  inlet_areas_AB=[.01, .01] m^2  inlet_heights_ABC=[.1, .05, 0] m  inlet_areas_ABC=[.01, .01, .01] m^2
      settings: SourceProductName=Simscape Fluids  SourceProductBaseCode=SH  InternalSimscapePortConfiguration="{\"Bottom\":[],\"Left\":[{\"id\":\"A\",\"label\":\"A\",\"type\":\"foundation.thermal_liquid.thermal_liquid\"}],\"Right\":[{\"id\":\"V_out\",\"label\":\"V\",\"type\":\"output\"},{\"id\":\"L_out\",\"label\":\"L\",\"type\":\"output\"},{\"id\":\"T_out\",\"label\":\"T\",\"type\":\"output\"},{\"id\":\"H\",\"label\":\"H\",\"type\":\"foundation.thermal.thermal\"}],\"Top\":[]}"
  Thermal Liquid Properties (TL) : SimscapeFluids_lib/Thermal Liquid/Utilities/Thermal Liquid Properties (TL)  Commented=on  fluid_list=fluids.thermal_liquid.utilities.enum.thermal_liquid_fluid_list.jet_A  concentration_param_EG=fluids.thermal_liquid.utilities.enum.thermal_liquid_concentration.volume_fraction  concentration_param_PG=fluids.thermal_liquid.utilities.enum.thermal_liquid_concentration.volume_fraction  c_mass_SW=3.5e-3  c_mass_EG=0.1  c_mass_PG=0.1  c_mass_GL=0.1  c_vol_EG=0.1  c_vol_PG=0.1  beta_const_EG=2.1791 GPa  beta_const_PG=2.1791 GPa  beta_const_GL=2.1791 GPa  p_min_EG=0.01 MPa  p_min_PG=0.01 MPa  p_min_GL=0.01 MPa  p_max_EG=50 MPa  p_max_PG=50 MPa  p_max_GL=50 MPa  p_atm=0.101325 MPa
      settings: SourceProductName=Simscape Fluids  SourceProductBaseCode=SH
  To LOX : SimscapeFluids_lib/Thermal Liquid/Tanks & Accumulators/Tank (TL)  Commented=on  pressure_spec=1  tank_pressure=0.101325 MPa  max_capacity=100 m^3  volume_spec=1  tank_area=3 m^2  level_TLU=[0, 3, 5] m  volume_TLU=[0, 4, 6] m^3  inlet_height=0.1 m  inlet_area=P_area in^2  g=9.81 m/s^2  level_specify=off  level_priority=Low  level=5 m  level_nominal_specify=off  level_nominal_unit=m  level_nominal_value=1  volume_specify=off  volume_priority=Low  volume=5 m^3  volume_nominal_specify=off  volume_nominal_unit=m^3  volume_nominal_value=1  mass_specify=off  mass_priority=Low  mass=5e+3 kg  mass_nominal_specify=off  mass_nominal_unit=kg  mass_nominal_value=1  T_tank_specify=off  T_tank_priority=Low  T_tank=293.15 K  T_tank_nominal_specify=off  T_tank_nominal_unit=K  T_tank_nominal_value=1  inlet_heights_AB=[.1, 0] m  inlet_areas_AB=[.01, .01] m^2  inlet_heights_ABC=[.1, .05, 0] m  inlet_areas_ABC=[.01, .01, .01] m^2
      settings: SourceProductName=Simscape Fluids  SourceProductBaseCode=SH  InternalSimscapePortConfiguration="{\"Bottom\":[],\"Left\":[{\"id\":\"A\",\"label\":\"A\",\"type\":\"foundation.thermal_liquid.thermal_liquid\"}],\"Right\":[{\"id\":\"V_out\",\"label\":\"V\",\"type\":\"output\"},{\"id\":\"L_out\",\"label\":\"L\",\"type\":\"output\"},{\"id\":\"T_out\",\"label\":\"T\",\"type\":\"output\"},{\"id\":\"H\",\"label\":\"H\",\"type\":\"foundation.thermal.thermal\"}],\"Top\":[]}"
  To RP-1 : SimscapeFluids_lib/Thermal Liquid/Tanks & Accumulators/Tank (TL)  Commented=on  pressure_spec=1  tank_pressure=0.101325 MPa  max_capacity=100 m^3  volume_spec=1  tank_area=3 m^2  level_TLU=[0, 3, 5] m  volume_TLU=[0, 4, 6] m^3  inlet_height=0.1 m  inlet_area=P_area in^2  g=9.81 m/s^2  level_specify=off  level_priority=Low  level=5 m  level_nominal_specify=off  level_nominal_unit=m  level_nominal_value=1  volume_specify=off  volume_priority=Low  volume=5 m^3  volume_nominal_specify=off  volume_nominal_unit=m^3  volume_nominal_value=1  mass_specify=off  mass_priority=Low  mass=5e+3 kg  mass_nominal_specify=off  mass_nominal_unit=kg  mass_nominal_value=1  T_tank_specify=off  T_tank_priority=Low  T_tank=293.15 K  T_tank_nominal_specify=off  T_tank_nominal_unit=K  T_tank_nominal_value=1  inlet_heights_AB=[.1, 0] m  inlet_areas_AB=[.01, .01] m^2  inlet_heights_ABC=[.1, .05, 0] m  inlet_areas_ABC=[.01, .01, .01] m^2
      settings: SourceProductName=Simscape Fluids  SourceProductBaseCode=SH  InternalSimscapePortConfiguration="{\"Bottom\":[],\"Left\":[{\"id\":\"A\",\"label\":\"A\",\"type\":\"foundation.thermal_liquid.thermal_liquid\"}],\"Right\":[{\"id\":\"V_out\",\"label\":\"V\",\"type\":\"output\"},{\"id\":\"L_out\",\"label\":\"L\",\"type\":\"output\"},{\"id\":\"T_out\",\"label\":\"T\",\"type\":\"output\"},{\"id\":\"H\",\"label\":\"H\",\"type\":\"foundation.thermal.thermal\"}],\"Top\":[]}"
  Valve Actuation Block : Subsystem  Commented=on
  Valve Actuation Block1 : Subsystem  Commented=on
  Valve Actuation Block10 : Subsystem  Commented=on
  Valve Actuation Block11 : Subsystem  Commented=on
  Valve Actuation Block2 : Subsystem  Commented=on
  Valve Actuation Block3 : Subsystem  Commented=on
  Valve Actuation Block4 : Subsystem  Commented=on
  Valve Actuation Block5 : Subsystem  Commented=on
  Valve Actuation Block6 : Subsystem  Commented=on
  Valve Actuation Block7 : Subsystem  Commented=on
  Valve Actuation Block8 : Subsystem  Commented=on
  Valve Actuation Block9 : Subsystem  Commented=on
  wires:
  Pressure input/1 -> Multiply/1
  PS-Simulink Converter6/1 -> Display4/1  "Volume"
  PS-Simulink Converter5/1 -> Display5/1  "Volume"
  Pressure input1/1 -> Simulink-PS Converter1/1
  From16/1 -> Valve Actuation Block3/1(Boolean signal)
  From18/1 -> Valve Actuation Block2/1(Boolean signal)
  From20/1 -> Valve Actuation Block6/1(Boolean signal)
  From21/1 -> Valve Actuation Block5/1(Boolean signal)
  From22/1 -> Valve Actuation Block8/1(Boolean signal)
  Pseudo input3/1(Scope) -> Input signal3/1
  From24/1 -> Valve Actuation Block10/1(Boolean signal)
  From25/1 -> Valve Actuation Block11/1(Boolean signal)
  Multiply/1 -> Display1/1, Simulink-PS Converter2/1
  Pseudo input1/1(Scope) -> Scope/2
  PS-Simulink Converter/1 -> Pressure Unit/1
  Pressure Unit/1 -> Scope/1
  From15/1 -> Valve Actuation Block1/1(Boolean signal)
  From17/1 -> Valve Actuation Block4/1(Boolean signal)
  From19/1 -> Valve Actuation Block7/1(Boolean signal)
  From23/1 -> Valve Actuation Block9/1(Boolean signal)
  From29/1 -> Final Pressures in the system/1
  From30/1 -> Final Pressures in the system/2
  From32/1 -> Final Volumes/2
  From31/1 -> Final Volumes/1
  PS-Simulink Converter1/1 -> Scope1/1  "Volume"
  PS-Simulink Converter2/1 -> Scope1/2  "Level"
  PS-Simulink Converter4/1 -> Scope1/4  "Temperature"
  PS-Simulink Converter3/1 -> Scope1/3  "Pressure"
  Pseudo input2/1(Scope) -> Scope2/1
  PS-Simulink Converter7/1 -> Scope2/2  "Pressure"
  PS-Simulink Converter8/1 -> Scope2/3  "Temperature"
  PS-Simulink Converter9/1 -> Scope3/1
  PS-Simulink Converter10/1 -> Scope3/2
  PS-Simulink Converter11/1 -> Scope4/1
  PS-Simulink Converter12/1 -> Scope4/2
  Ramp/1 -> Saturation/1
  Saturation/1 -> Simulink-PS Converter/1, Scope5/1
  connections:
  Pressure Relief Valve (TL)1/LConn1 -- RP-1 Tank/RConn1 -- Subsystem6/LConn1 -- F-EV-2/LConn1 -- Pipe (TL)1/LConn1 -- Subsystem4/LConn1
  Pipe (TL)1/RConn1 -- Subsystem5/LConn1 -- F-EV-3/LConn1
  Perfect Insulator4/LConn1 -- Pipe (TL)1/LConn2
  Reservoir (TL)1/LConn1 -- Pressure Relief Valve (TL)1/RConn1
  Simulink-PS Converter2/RConn1 -- RP-1 Tank/LConn1
  PS-Simulink Converter6/LConn1 -- To LOX/RConn1 -- Engine Inlet Parameters4/LConn1
  To LOX/RConn3 -- Engine Inlet Parameters4/LConn3
  Perfect Insulator6/LConn1 -- To LOX/RConn4
  To LOX/RConn2 -- Engine Inlet Parameters4/LConn2
  P-EV-1/RConn1 -- Reservoir (TL)9/LConn1
  Pressurant Tank/RConn1 -- P-EV-2/LConn1 -- Subsystem7/LConn1 -- P-EV-1/LConn1
  P-EV-2/RConn1 -- P-EV-4/LConn1 -- Pressure Relief Valve (TL)3/LConn1 -- P-EV-5/LConn1 -- Subsystem8/LConn1 -- Pressure Relief Valve (TL)/LConn1 -- Subsystem9/LConn1 -- P-EV-3/LConn1
  Engine Inlet Parameters5/LConn1 -- To RP-1/RConn1 -- PS-Simulink Converter5/LConn1
  P-EV-5/RConn1 -- To RP-1/LConn1 -- F-EV-1/LConn1
  To RP-1/RConn2 -- Engine Inlet Parameters5/LConn2
  To RP-1/RConn3 -- Engine Inlet Parameters5/LConn3
  Perfect Insulator7/LConn1 -- To RP-1/RConn4
  Solver Configuration3/RConn1 -- P-EV-3/RConn1 -- To LOX/LConn1 -- O-SV-1/LConn1
  Reservoir (TL)2/LConn1 -- O-SV-1/RConn1
  Reservoir (TL)3/LConn1 -- F-EV-1/RConn1
  Solver Configuration1/RConn1 -- Combustion Chamber/LConn1 -- LOX Final/LConn1 -- O-EV-3/RConn1
  Combustion Chamber/LConn2 -- F-EV-3/RConn1 -- RP1 Final/LConn1 -- Solver Configuration2/RConn1
  F-EV-2/RConn1 -- Reservoir (TL)4/LConn1
  Pressure Relief Valve (TL)2/LConn1 -- Subsystem1/LConn1 -- Pipe (TL)2/LConn1 -- Subsystem3/LConn1 -- O-EV-1/LConn1 -- LOX Tank/RConn1
  Subsystem2/LConn1 -- O-EV-3/LConn1 -- Pipe (TL)2/RConn1
  O-EV-1/RConn1 -- Reservoir (TL)6/LConn1
  Reservoir (TL)5/LConn1 -- Pressure Relief Valve (TL)2/RConn1
  Simulink-PS Converter1/RConn1 -- LOX Tank/LConn1
  Perfect Insulator1/LConn1 -- Pipe (TL)2/LConn2
  Reservoir (TL)/LConn1 -- Pressure Relief Valve (TL)/RConn1
  Reservoir (TL)7/LConn1 -- P-EV-4/RConn1
  Reservoir (TL)8/LConn1 -- Pressure Relief Valve (TL)3/RConn1
  Valve Actuation Block2/RConn1 -- P-EV-2/LConn2
  O-SV-1/LConn2 -- Valve Actuation Block6/RConn1
  Valve Actuation Block5/RConn1 -- F-EV-1/LConn2
  Valve Actuation Block8/RConn1 -- O-EV-1/LConn2
  Valve Actuation Block10/RConn1 -- F-EV-3/LConn2
  F-EV-2/LConn2 -- Valve Actuation Block11/RConn1
  P-EV-6/RConn1 -- Tank (TL)/LConn1 -- Solver Configuration/RConn1 -- Subsystem10/LConn1
  P-EV-6/LConn1 -- Pressurant Tank1/RConn1
  Pseudo input1/RConn1 -- P-EV-6/LConn2
  Subsystem10/RConn1 -- PS-Simulink Converter/LConn1
  Valve Actuation Block1/RConn1 -- P-EV-1/LConn2
  Valve Actuation Block3/RConn1 -- P-EV-4/LConn2
  Valve Actuation Block4/RConn1 -- P-EV-5/LConn2
  Valve Actuation Block7/RConn1 -- P-EV-3/LConn2
  Valve Actuation Block9/RConn1 -- O-EV-3/LConn2
  Pressure Source (G)/LConn1 -- Pressure & Temperature Sensor (G)/LConn1 -- Reservoir (G)/LConn1
  Local Restriction (G)/LConn1 -- Pressure Source (G)/RConn1
  Reservoir (TL)10/LConn1 -- Pressure Source (TL)/LConn1
  Local Restriction (G)/RConn1 -- Solver Configuration4/RConn1 -- Pressure & Temperature Sensor (G)1/LConn1 -- Tank (G-TL)/LConn1
  Reservoir (G)1/LConn1 -- Pressure Relief Valve (G)/RConn1
  Perfect Insulator/LConn1 -- Tank (G-TL)/RConn1
  Tank (G-TL)/RConn2 -- Perfect Insulator2/LConn1
  PS-Simulink Converter1/LConn1 -- Tank (G-TL)/RConn3
  PS-Simulink Converter2/LConn1 -- Tank (G-TL)/RConn4
  Pressure Relief Valve (G)/LConn1 -- Tank (G-TL)/LConn2
  Pressure & Temperature Sensor (G)/RConn2 -- PS-Simulink Converter3/LConn1
  Pressure & Temperature Sensor (G)/RConn3 -- PS-Simulink Converter4/LConn1
  Reservoir (G)2/LConn1 -- Pressure & Temperature Sensor (G)/RConn1
  Pseudo input2/RConn1 -- Local Restriction (G)/LConn2
  Reservoir (G)3/LConn1 -- Pressure & Temperature Sensor (G)1/RConn1
  Pressure & Temperature Sensor (G)1/RConn2 -- PS-Simulink Converter7/LConn1
  Pressure & Temperature Sensor (G)1/RConn3 -- PS-Simulink Converter8/LConn1
  Pressure Source (TL)/RConn1 -- Tank (G-TL)/LConn3
  Reservoir (G)4/LConn1 -- Solver Configuration5/RConn1 -- Pressure Source (G)1/LConn1
  Pressure & Temperature Sensor (G)2/LConn1 -- Local Restriction (G)1/LConn1 -- Pressure Source (G)1/RConn1
  Pressure & Temperature Sensor (G)2/RConn1 -- Reservoir (G)5/LConn1
  Tank (G-TL)1/LConn1 -- Pressure & Temperature Sensor (G)3/LConn1 -- Local Restriction (G)1/RConn1
  Tank (G-TL)1/RConn1 -- Perfect Insulator3/LConn1
  Tank (G-TL)1/RConn2 -- Perfect Insulator5/LConn1
  Tank (G-TL)1/RConn3 -- PS-Simulink Converter9/LConn1
  Tank (G-TL)1/RConn4 -- PS-Simulink Converter10/LConn1
  Reservoir (G)6/LConn1 -- Infinite Flow Resistance (G)/RConn1
  Tank (G-TL)1/LConn3 -- Reservoir (TL)11/LConn1
  Pressure & Temperature Sensor (G)2/RConn3 -- PS Terminator/LConn1
  Pressure & Temperature Sensor (G)2/RConn2 -- PS-Simulink Converter11/LConn1
  Pressure & Temperature Sensor (G)3/RConn1 -- Reservoir (G)7/LConn1
  PS-Simulink Converter12/LConn1 -- Pressure & Temperature Sensor (G)3/RConn2
  PS Terminator1/LConn1 -- Pressure & Temperature Sensor (G)3/RConn3
  Simulink-PS Converter/RConn1 -- Local Restriction (G)1/LConn2
  Infinite Flow Resistance (G)/LConn1 -- Tank (G-TL)1/LConn2
